simulink model "s_ehiga_low_gain_control"  (R2020a)
settings: Solver=ode1  StartTime=0.0  StopTime=200  FixedStep=0.002  RelTol=1e-3  EnableMultiTasking=on
undefined symbols (not defined in the file or in its folder): A, B, C, D, G
libraries: simulink_extras x4, quarc_library x3
settings Model: ExtModeTrigDuration=10000  Creator=ehiga  LastModifiedBy=ehiga
settings SolverCC: PositivePriorityOrder=on
settings DataIOCC: ReturnWorkspaceOutputs=off
settings OptimizationCC: LifeSpan=inf
settings DebuggingCC: ArithmeticOperatorsInVariantConditions=warning
settings SFSimCC: SimUseLocalCustomCode=off  CustomCodeUndefinedFunction=UseInterfaceOnly
settings RTWCC: Description=QUARC Win64 Target  SystemTargetFile=quarc_win64.tlc  TemplateMakefile=quarc_default_tmf  RTWUseLocalCustomCode=off
settings CodeAppCC: StateflowObjectComments=on
settings STFCustomTargetCC: TargetPreCompLibLocation=C:\PROGRA~3\QUARC\lib\2020a\win64\release  TargetLangStandard=C99 (ISO)  ConcurrentExecutionCompliant=on  GRTInterface=on  SystemTargetFile=quarc_win64.tlc
settings GRTTargetCC: TargetPreCompLibLocation=C:\PROGRA~3\QUARC\lib\2020a\win64\release  ParMdlRefBuildCompliant=off  CompOptLevelCompliant=off  CombineOutputUpdateFcns=off  MatFileLogging=off  CPPClassGenCompliant=off  GRTInterface=on  UseToolchainInfoCompliant=off  ExtMode=on  ExtModeMexFile=quarc_comm
settings ConfigComp: CovMetricSettings=dswe

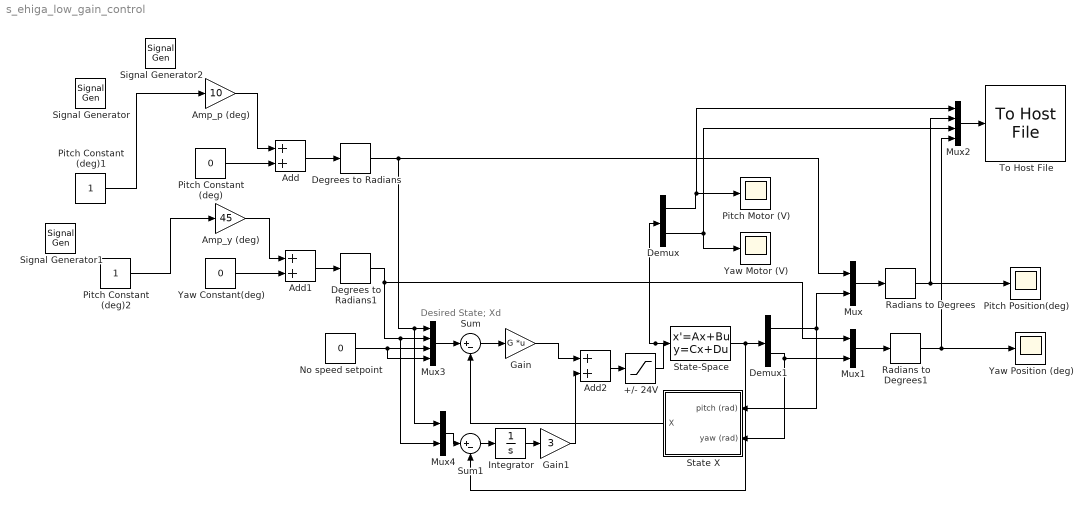
== system s_ehiga_low_gain_control ==
  note: Desired State; Xd
  +/- 24V : Saturate  UpperLimit=24  LowerLimit=-24
  Add : Sum
  Add1 : Sum
  Add2 : Sum
  Amp_p (deg) : Gain  Gain=10
  Amp_y (deg) : Gain  Gain=45
  Degrees to Radians : simulink_extras/Transformations/Degrees to Radians
  Degrees to Radians1 : simulink_extras/Transformations/Degrees to Radians
  Demux : Demux  Outputs=2
  Demux1 : Demux  Outputs=2
  Gain : Gain  Gain=G  Multiplication=Matrix(K*u)
  Gain1 : Gain  Gain=3
  Integrator : Integrator
  Mux : Mux  Inputs=2
  Mux1 : Mux  Inputs=2
  Mux2 : Mux
  Mux3 : Mux
  Mux4 : Mux  Inputs=2
  No speed setpoint : Constant  Value=0
  Pitch Constant (deg) : Constant  Value=0
  Pitch Constant (deg)1 : Constant
  Pitch Constant (deg)2 : Constant
  Pitch Motor (V) : Scope
  Pitch Position(deg) : Scope
  Radians to Degrees : simulink_extras/Transformations/Radians to Degrees
  Radians to Degrees1 : simulink_extras/Transformations/Radians to Degrees
  Signal Generator : SignalGenerator  WaveForm=square  Frequency=0.1
  Signal Generator1 : SignalGenerator  WaveForm=square  Frequency=0.04
  Signal Generator2 : SignalGenerator  WaveForm=square  Frequency=0.06
  State X : Subsystem
  State-Space : StateSpace  A=A  B=B  C=C  D=D  InitialCondition=0
  Sum : Sum  Inputs=|+-
  Sum1 : Sum  Inputs=|+-
  To Host File : quarc_library/Sinks/To Host/To Host File  file_name=aero_lqr_rsp_sim.mat  variable_name=lqr_rsp_sim  decimation=1  sample_time=-1  file_format=MAT-file v.4  options=No header or footer  append=off  final_file_name=aero_lqr_rsp_sim.mat  bitrate=2000000
  Yaw Constant(deg) : Constant  Value=0
  Yaw Motor (V) : Scope
  Yaw Position (deg) : Scope
  wires:
  Degrees to Radians1/1 -> Mux4/2, Mux3/2, Mux1/1
  Demux1/2 -> Mux1/2, State X/2(yaw (rad))
  Mux2/1 -> To Host File/1
  Mux3/1 -> Sum/1
  State-Space/1 -> Sum1/2, Demux1/1
  Add/1 -> Degrees to Radians/1
  Pitch Constant (deg)/1 -> Add/2
  Demux1/1 -> Mux/2, State X/1(pitch (rad))
  No speed setpoint/1 -> Mux3/4, Mux3/3
  Mux1/1 -> Radians to Degrees1/1
  Sum/1 -> Gain/1
  Radians to Degrees1/1 -> Mux2/4, Yaw Position (deg)/1
  +/- 24V/1 -> Demux/1, State-Space/1
  Demux/1 -> Mux2/1, Pitch Motor (V)/1
  Degrees to Radians/1 -> Mux4/1, Mux3/1, Mux/1
  State X/1(X) -> Sum/2
  Amp_p (deg)/1 -> Add/1
  Radians to Degrees/1 -> Mux2/2, Pitch Position(deg)/1
  Yaw Constant(deg)/1 -> Add1/2
  Demux/2 -> Yaw Motor (V)/1, Mux2/3
  Mux/1 -> Radians to Degrees/1
  Add1/1 -> Degrees to Radians1/1
  Amp_y (deg)/1 -> Add1/1
  Mux4/1 -> Sum1/1
  Gain/1 -> Add2/1
  Add2/1 -> +/- 24V/1
  Sum1/1 -> Integrator/1
  Integrator/1 -> Gain1/1
  Gain1/1 -> Add2/2
  Pitch Constant (deg)1/1 -> Amp_p (deg)/1
  Pitch Constant (deg)2/1 -> Amp_y (deg)/1

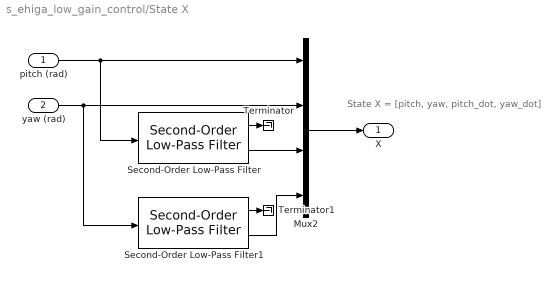
== system s_ehiga_low_gain_control/State X ==
  note: State X = [pitch, yaw, pitch_dot, yaw_dot]
  pitch (rad) : Inport
  yaw (rad) : Inport  Port=2
  Mux2 : Mux
  Second-Order Low-Pass Filter : quarc_library/Continuous/Second-Order Low-Pass Filter  params_source=Internal (dialog parameters)  input_width=50  input_zeta=0.8  input_init=0
  Second-Order Low-Pass Filter1 : quarc_library/Continuous/Second-Order Low-Pass Filter  params_source=Internal (dialog parameters)  input_width=50  input_zeta=0.8  input_init=0
  Terminator : Terminator
  Terminator1 : Terminator
  X : Outport
  wires:
  Mux2/1 -> X/1
  yaw (rad)/1 -> Second-Order Low-Pass Filter1/1, Mux2/2
  pitch (rad)/1 -> Second-Order Low-Pass Filter/1, Mux2/1
  Second-Order Low-Pass Filter/2 -> Mux2/3
  Second-Order Low-Pass Filter1/2 -> Mux2/4
  Second-Order Low-Pass Filter/1 -> Terminator/1
  Second-Order Low-Pass Filter1/1 -> Terminator1/1
